simulink model "MPCFollower"  (R2024a)
settings: Solver=FixedStepAuto  StartTime=0.0  StopTime=inf  RelTol=1e-3
undefined symbols (not defined in the file or in its folder): maxLocalPathLen, maxRefPathLen, nlobjTracking
libraries: roshelperlib x2, mpclib x1
settings Model: Creator=cstabile  LastModifiedBy=cstabile

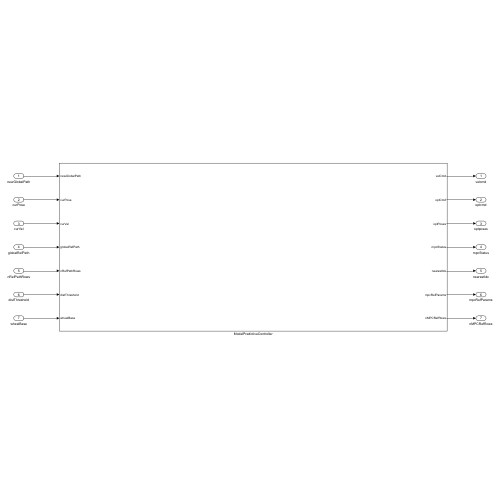
[thumbnail: Simulink's stored preview of the top-level diagram]
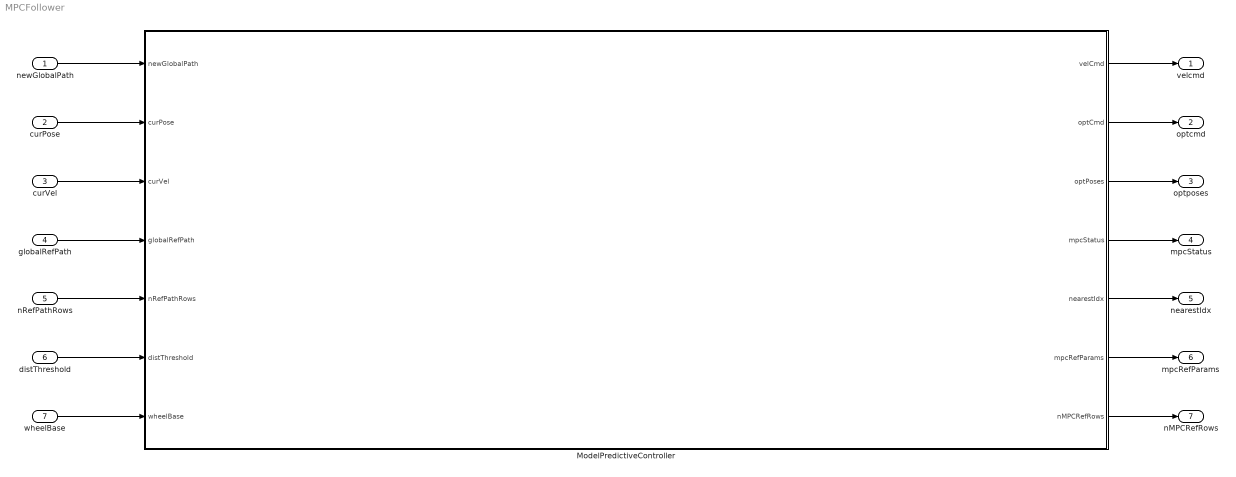
== system MPCFollower ==
  newGlobalPath : Inport  PortDimensions=1
  curPose : Inport  Port=2  PortDimensions=[1 3]
  curVel : Inport  Port=3  PortDimensions=[1 2]
  globalRefPath : Inport  Port=4  PortDimensions=[maxRefPathLen 3]
  nRefPathRows : Inport  Port=5
  distThreshold : Inport  Port=6
  wheelBase : Inport  Port=7
  ModelPredictiveController : Subsystem
  velcmd : Outport  PortDimensions=[1 2]
  optcmd : Outport  Port=2  PortDimensions=[nlobjTracking.PredictionHorizon+1 2]
  optposes : Outport  Port=3  PortDimensions=[nlobjTracking.PredictionHorizon+1 3]
  mpcStatus : Outport  Port=4
  nearestIdx : Outport  Port=5
  mpcRefParams : Outport  Port=6  PortDimensions=[nlobjTracking.PredictionHorizon 3]
  nMPCRefRows : Outport  Port=7  PortDimensions=1
  wires:
  newGlobalPath/1 -> ModelPredictiveController/1(newGlobalPath)
  curPose/1 -> ModelPredictiveController/2(curPose)
  ModelPredictiveController/1(velCmd) -> velcmd/1
  distThreshold/1 -> ModelPredictiveController/6(distThreshold)
  curVel/1 -> ModelPredictiveController/3(curVel)
  globalRefPath/1 -> ModelPredictiveController/4(globalRefPath)
  nRefPathRows/1 -> ModelPredictiveController/5(nRefPathRows)
  wheelBase/1 -> ModelPredictiveController/7(wheelBase)
  ModelPredictiveController/3(optPoses) -> optposes/1
  ModelPredictiveController/2(optCmd) -> optcmd/1
  ModelPredictiveController/5(nearestIdx) -> nearestIdx/1
  ModelPredictiveController/4(mpcStatus) -> mpcStatus/1
  ModelPredictiveController/6(mpcRefParams) -> mpcRefParams/1
  ModelPredictiveController/7(nMPCRefRows) -> nMPCRefRows/1

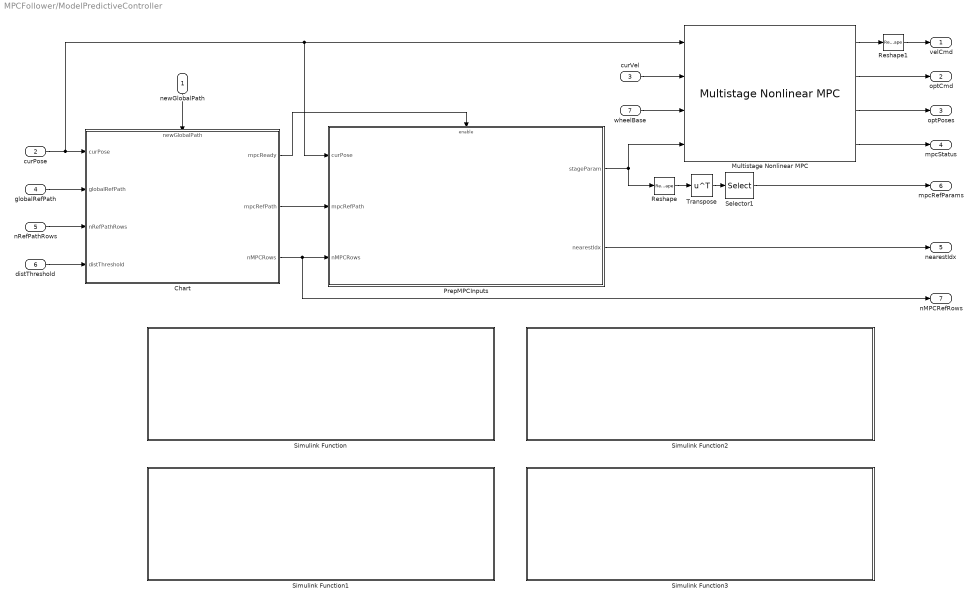
== system MPCFollower/ModelPredictiveController ==
  newGlobalPath : Inport
  curPose : Inport  Port=2  PortDimensions=[1 3]
  curVel : Inport  Port=3
  globalRefPath : Inport  Port=4  PortDimensions=[maxRefPathLen 3]
  nRefPathRows : Inport  Port=5
  distThreshold : Inport  Port=6
  wheelBase : Inport  Port=7
  Chart : Stateflow chart  TreatAsAtomicUnit=on
      settings: PortSchema="{\"entries\":[{\"content\":{\"sides\":[{\"content\":{\"connectorIds\":[\"In2\",\"In3\",\"In4\",\"In5\"]},\"type\":\"ConnectorPlacement.EquallySpacedRectSide\",\"uuid\":\"d330c18e-78c4-4446-bef4-6c07f5901eab\"},{\"content\":{\"connectorIds\":[\"Out1\",\"Out2\",\"Out3\"],\"side\":\"RIGHT\"},\"type\":\"ConnectorPlacement.EquallySpacedRectSide\",\"uuid\":\"b290a02e-6c58-4d00-b488-7afeab83322a\"},{\"content\":{\"connectorIds\":[\"In1\"],\"side\":\"TOP\"},\"type\":\"ConnectorPlacement.EquallySpacedRectSide\",\"uuid\":\"5cf05c0e-e546-4e08-b885-e292e35119c9\"}]},\"type\":\"ConnectorPlacement.EquallySpacedConnector\",\"uuid\":\"c70a4d9b-d7d3-4706-8fc9-b9f30a67664a\"}],\"packageUris\":[\"http://schema.mathworks.com/mf0/Connector/R2020b\"],\"version\":\"1.0\"}"
  Multistage Nonlinear MPC : mpclib/Multistage Nonlinear MPC  nlmpcobj=nlobjTracking  UseObjectTs=on  TsControl=-1  UseMEX=off  mexname=pathFollowingMPCMex  md_enabled=off  stateparam_enabled=on  stageparam_enabled=on  cost_enabled=off  mvseq_enabled=on  stateseq_enabled=on  slack_enabled=off  status_enabled=on  mv_min=off  mv_max=off  mvrate_min=off  mvrate_max=off  state_min=off  state_max=off  terminal_state=off  nlp_initialize=off
  PrepMPCInputs : Subsystem
  Reshape : Reshape  OutputDimensionality=Customize  OutputDimensions=[4,11]
  Reshape1 : Reshape  OutputDimensionality=Row vector (2-D)
  Selector1 : Selector  NumberOfDimensions=2  InputPortWidth=3  IndexOptions=Index vector (dialog),Index vector (dialog)  Indices=2:11,1:3  OutputSizes=1,1
  Simulink Function : Subsystem  TreatAsAtomicUnit=on
  Simulink Function1 : Subsystem  TreatAsAtomicUnit=on
  Simulink Function2 : Subsystem  TreatAsAtomicUnit=on
  Simulink Function3 : Subsystem  TreatAsAtomicUnit=on
  Transpose : Math  Operator=transpose
  velCmd : Outport  PortDimensions=[1 2]
  optCmd : Outport  Port=2
  optPoses : Outport  Port=3
  mpcStatus : Outport  Port=4
  nearestIdx : Outport  Port=5
  mpcRefParams : Outport  Port=6
  nMPCRefRows : Outport  Port=7
  wires:
  curPose/1 -> Multistage Nonlinear MPC/1, PrepMPCInputs/1(curPose), Chart/2(curPose)
  wheelBase/1 -> Multistage Nonlinear MPC/3
  Multistage Nonlinear MPC/2 -> optCmd/1
  Multistage Nonlinear MPC/1 -> Reshape1/1
  distThreshold/1 -> Chart/5(distThreshold)
  Multistage Nonlinear MPC/3 -> optPoses/1
  Multistage Nonlinear MPC/4 -> mpcStatus/1
  curVel/1 -> Multistage Nonlinear MPC/2
  globalRefPath/1 -> Chart/3(globalRefPath)
  nRefPathRows/1 -> Chart/4(nRefPathRows)
  Reshape/1 -> Transpose/1
  Transpose/1 -> Selector1/1
  Selector1/1 -> mpcRefParams/1
  newGlobalPath/1 -> Chart/1(newGlobalPath)
  PrepMPCInputs/1(stageParam) -> Reshape/1, Multistage Nonlinear MPC/4
  Chart/2(mpcRefPath) -> PrepMPCInputs/2(mpcRefPath)
  Chart/3(nMPCRows) -> nMPCRefRows/1, PrepMPCInputs/3(nMPCRows)
  PrepMPCInputs/2(nearestIdx) -> nearestIdx/1
  Chart/1(mpcReady) -> PrepMPCInputs/Enable
  Reshape1/1 -> velCmd/1

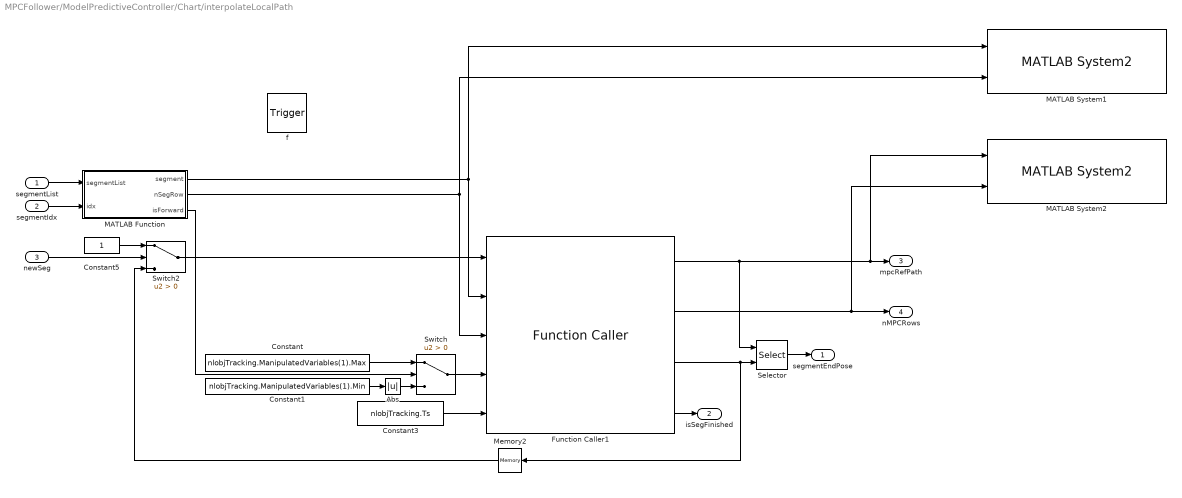
== system MPCFollower/ModelPredictiveController/Chart/interpolateLocalPath ==
  segmentList : Inport  OutDataTypeStr=Bus: mpcPathList_fixed_bus  PortDimensions=1
  segmentIdx : Inport  Port=2  OutDataTypeStr=double  PortDimensions=1
  newSeg : Inport  Port=3  OutDataTypeStr=boolean  PortDimensions=1
  f : TriggerPort  TriggerType=function-call  VariantControl=(inherit)
      settings: CopyFcn=Stateflow.SLINSF.SimulinkMan.removeBlockPreDeleteFcn  PreDeleteFcn=Stateflow.SLINSF.SimulinkMan.unsafePredeleteFcn
  Abs : Abs  SaturateOnIntegerOverflow=off
  Constant : Constant  Value=nlobjTracking.ManipulatedVariables(1).Max
  Constant1 : Constant  Value=nlobjTracking.ManipulatedVariables(1).Min
  Constant3 : Constant  Value=nlobjTracking.Ts
  Constant5 : Constant
  Function Caller1 : FunctionCaller  FunctionPrototype=[localRefPath,nRows,lastIdx,isSegFinished] = arcInterpolateSegment(initIdx,segmentPoses,nSegRows,vNominal,timestep)  InputArgumentSpecifications=<Enter example>  OutputArgumentSpecifications=<Enter example>
  MATLAB Function : MATLAB Function  TreatAsAtomicUnit=on
  MATLAB System1 : roshelperlib/MATLAB System2  VisualizationParameters={'m','LineWidth',4}  PlotType=Line  DisplayVisual=on  SimulateUsing=Interpreted execution
  MATLAB System2 : roshelperlib/MATLAB System2  VisualizationParameters={'r:','LineWidth',3}  PlotType=Line  DisplayVisual=on  SimulateUsing=Interpreted execution
  Memory2 : Memory  InheritSampleTime=on
  Selector : Selector  NumberOfDimensions=2  InputPortWidth=3  IndexOptions=Index vector (port),Select all  Indices=[1 3],1  OutputSizes=1,1
  Switch : Switch  Criteria=u2 > Threshold  SaturateOnIntegerOverflow=off  InputSameDT=off
  Switch2 : Switch  Criteria=u2 > Threshold  SaturateOnIntegerOverflow=off  InputSameDT=off
  segmentEndPose : Outport
  isSegFinished : Outport  Port=2
  mpcRefPath : Outport  Port=3
  nMPCRows : Outport  Port=4
  wires:
  Switch2/1 -> Function Caller1/1
  Constant1/1 -> Abs/1
  Function Caller1/2 -> MATLAB System2/2, nMPCRows/1
  Function Caller1/3 -> Selector/2, Memory2/1
  Constant/1 -> Switch/1
  Switch/1 -> Function Caller1/4
  Selector/1 -> segmentEndPose/1
  Function Caller1/4 -> isSegFinished/1
  segmentList/1 -> MATLAB Function/1(segmentList)
  MATLAB Function/2(nSegRow) -> Function Caller1/3, MATLAB System1/2
  Constant5/1 -> Switch2/1
  segmentIdx/1 -> MATLAB Function/2(idx)
  MATLAB Function/3(isForward) -> Switch/2
  Constant3/1 -> Function Caller1/5
  Function Caller1/1 -> MATLAB System2/1, mpcRefPath/1, Selector/1
  MATLAB Function/1(segment) -> Function Caller1/2, MATLAB System1/1
  Memory2/1 -> Switch2/3
  newSeg/1 -> Switch2/2
  Abs/1 -> Switch/3

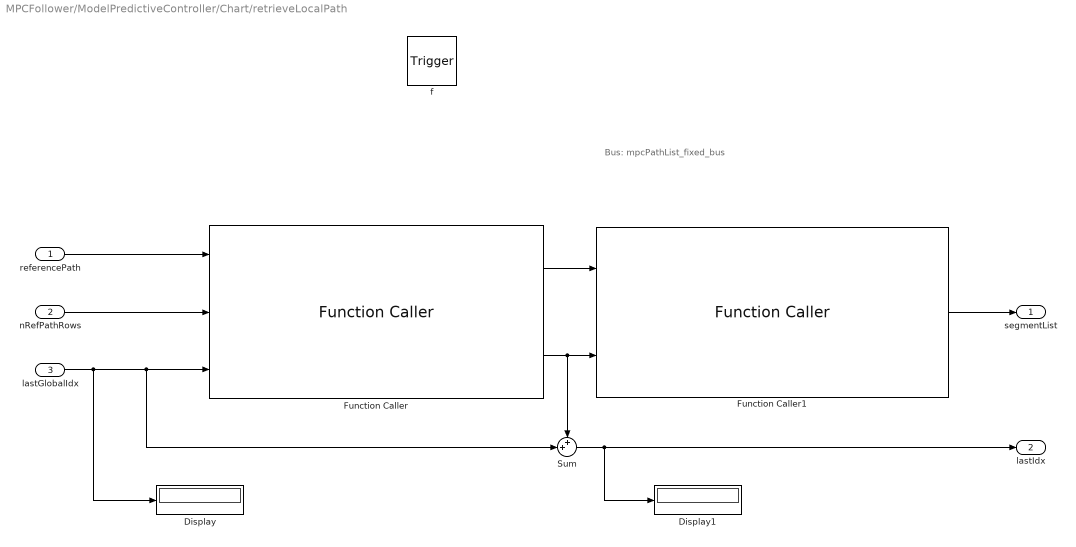
== system MPCFollower/ModelPredictiveController/Chart/retrieveLocalPath ==
  note: Bus: mpcPathList_fixed_bus
  referencePath : Inport  OutDataTypeStr=double  PortDimensions=[maxRefPathLen 3]
  nRefPathRows : Inport  Port=2  OutDataTypeStr=double  PortDimensions=1
  lastGlobalIdx : Inport  Port=3  OutDataTypeStr=double  PortDimensions=1
  f : TriggerPort  TriggerType=function-call  VariantControl=(inherit)
      settings: CopyFcn=Stateflow.SLINSF.SimulinkMan.removeBlockPreDeleteFcn  PreDeleteFcn=Stateflow.SLINSF.SimulinkMan.unsafePredeleteFcn
  Display : Display
  Display1 : Display
  Function Caller : FunctionCaller  FunctionPrototype=[localRefPath,nLocalRows] = getLocalPath(referencePath,nRefPathRows,curGlobalIdx)  InputArgumentSpecifications=<Enter example>  OutputArgumentSpecifications=<Enter example>
  Function Caller1 : FunctionCaller  FunctionPrototype=segmentList = path2segments(referencePath,nLocalRows)  InputArgumentSpecifications=<Enter example>  OutputArgumentSpecifications=<Enter example>
  Sum : Sum  Inputs=++|
  segmentList : Outport  OutDataTypeStr=Bus: mpcPathList_fixed_bus  PortDimensions=1
  lastIdx : Outport  Port=2  OutDataTypeStr=double  PortDimensions=1
  wires:
  lastGlobalIdx/1 -> Display/1, Sum/2, Function Caller/3
  Function Caller/1 -> Function Caller1/1
  nRefPathRows/1 -> Function Caller/2
  referencePath/1 -> Function Caller/1
  Function Caller/2 -> Sum/1, Function Caller1/2
  Sum/1 -> Display1/1, lastIdx/1
  Function Caller1/1 -> segmentList/1

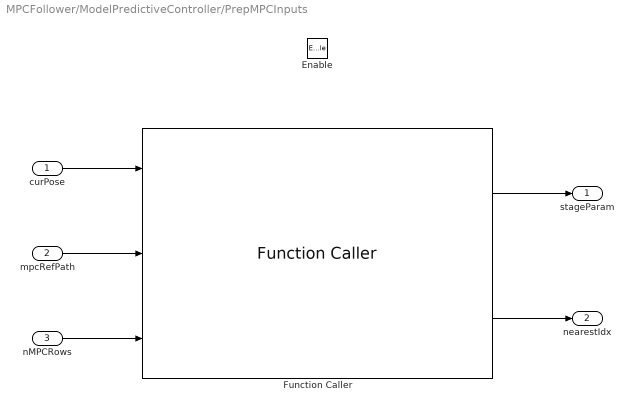
== system MPCFollower/ModelPredictiveController/PrepMPCInputs ==
  curPose : Inport
  mpcRefPath : Inport  Port=2
  nMPCRows : Inport  Port=3
  Enable : EnablePort  StatesWhenEnabling=reset
  Function Caller : FunctionCaller  FunctionPrototype=[stageParam,idx] = generateMPCReferenceStates(curPose,refPath,nRefPathRows)  InputArgumentSpecifications=<Enter example>  OutputArgumentSpecifications=<Enter example>
  stageParam : Outport
  nearestIdx : Outport  Port=2
  wires:
  Function Caller/1 -> stageParam/1
  nMPCRows/1 -> Function Caller/3
  curPose/1 -> Function Caller/1
  mpcRefPath/1 -> Function Caller/2
  Function Caller/2 -> nearestIdx/1

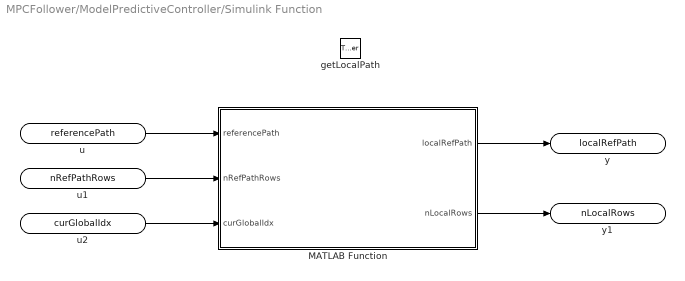
== system MPCFollower/ModelPredictiveController/Simulink Function ==
  getLocalPath : TriggerPort  TriggerType=function-call  IsSimulinkFunction=on  FunctionName=getLocalPath  VariantControl=(inherit)
  MATLAB Function : MATLAB Function  TreatAsAtomicUnit=on  mask{maxPathLength=maxRefPathLen, maxLocalLength=maxLocalPathLen}
      mask prompts: maxPathLength "Max Path Length"; maxLocalLength "Max Local Path Length"
  u : ArgIn  DisableCoverage=on  PortDimensions=[maxRefPathLen 3]  ArgumentName=referencePath
  u1 : ArgIn  DisableCoverage=on  Port=2  ArgumentName=nRefPathRows
  u2 : ArgIn  DisableCoverage=on  Port=3  ArgumentName=curGlobalIdx
  y : ArgOut  DisableCoverage=on  PortDimensions=[maxLocalPathLen 3]  ArgumentName=localRefPath
  y1 : ArgOut  DisableCoverage=on  Port=2  ArgumentName=nLocalRows
  wires:
  MATLAB Function/1(localRefPath) -> y/1
  MATLAB Function/2(nLocalRows) -> y1/1
  u/1 -> MATLAB Function/1(referencePath)
  u2/1 -> MATLAB Function/3(curGlobalIdx)
  u1/1 -> MATLAB Function/2(nRefPathRows)

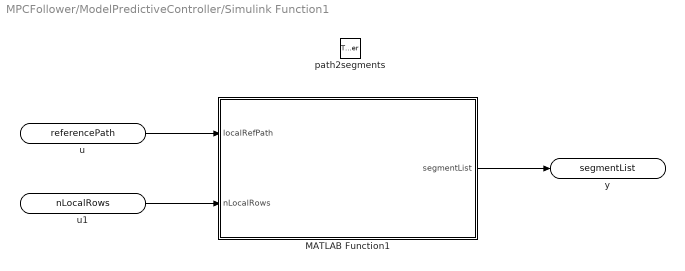
== system MPCFollower/ModelPredictiveController/Simulink Function1 ==
  path2segments : TriggerPort  TriggerType=function-call  IsSimulinkFunction=on  FunctionName=path2segments  VariantControl=(inherit)
  MATLAB Function1 : MATLAB Function  TreatAsAtomicUnit=on  mask{maxPathLength=maxRefPathLen, maxLocalLength=maxLocalPathLen}
      mask prompts: maxPathLength "Max Path Length"; maxLocalLength "Max Local Path Length"
  u : ArgIn  DisableCoverage=on  PortDimensions=[maxLocalPathLen 3]  ArgumentName=referencePath
  u1 : ArgIn  DisableCoverage=on  Port=2  ArgumentName=nLocalRows
  y : ArgOut  DisableCoverage=on  OutDataTypeStr=Bus: mpcPathList_fixed_bus  ArgumentName=segmentList
  wires:
  MATLAB Function1/1(segmentList) -> y/1
  u/1 -> MATLAB Function1/1(localRefPath)
  u1/1 -> MATLAB Function1/2(nLocalRows)

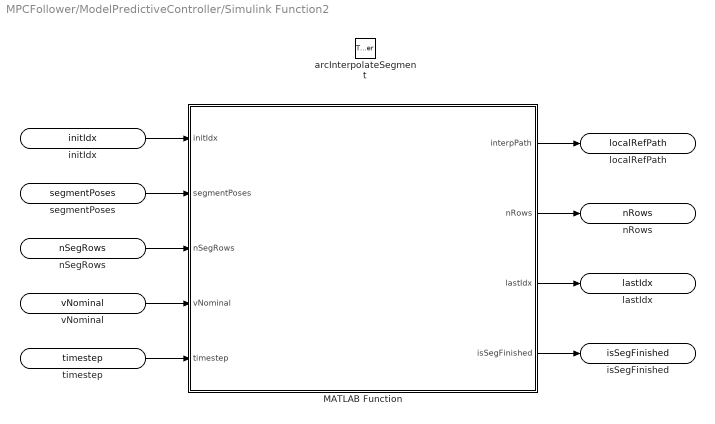
== system MPCFollower/ModelPredictiveController/Simulink Function2 ==
  arcInterpolateSegment : TriggerPort  TriggerType=function-call  IsSimulinkFunction=on  FunctionName=arcInterpolateSegment  VariantControl=(inherit)
  MATLAB Function : MATLAB Function  TreatAsAtomicUnit=on  mask{maxPathLength=maxLocalPathLen}
      mask prompts: maxPathLength "Max Path Length"
  initIdx : ArgIn  DisableCoverage=on  ArgumentName=initIdx
  segmentPoses : ArgIn  DisableCoverage=on  Port=2  PortDimensions=[maxLocalPathLen 3]  ArgumentName=segmentPoses
  nSegRows : ArgIn  DisableCoverage=on  Port=3  ArgumentName=nSegRows
  vNominal : ArgIn  DisableCoverage=on  Port=4  ArgumentName=vNominal
  timestep : ArgIn  DisableCoverage=on  Port=5  ArgumentName=timestep
  localRefPath : ArgOut  DisableCoverage=on  PortDimensions=[maxLocalPathLen 3]  ArgumentName=localRefPath
  nRows : ArgOut  DisableCoverage=on  Port=2  ArgumentName=nRows
  lastIdx : ArgOut  DisableCoverage=on  Port=3  ArgumentName=lastIdx
  isSegFinished : ArgOut  DisableCoverage=on  Port=4  OutDataTypeStr=boolean  ArgumentName=isSegFinished
  wires:
  segmentPoses/1 -> MATLAB Function/2(segmentPoses)
  initIdx/1 -> MATLAB Function/1(initIdx)
  vNominal/1 -> MATLAB Function/4(vNominal)
  timestep/1 -> MATLAB Function/5(timestep)
  MATLAB Function/1(interpPath) -> localRefPath/1
  MATLAB Function/3(lastIdx) -> lastIdx/1
  MATLAB Function/4(isSegFinished) -> isSegFinished/1
  MATLAB Function/2(nRows) -> nRows/1
  nSegRows/1 -> MATLAB Function/3(nSegRows)

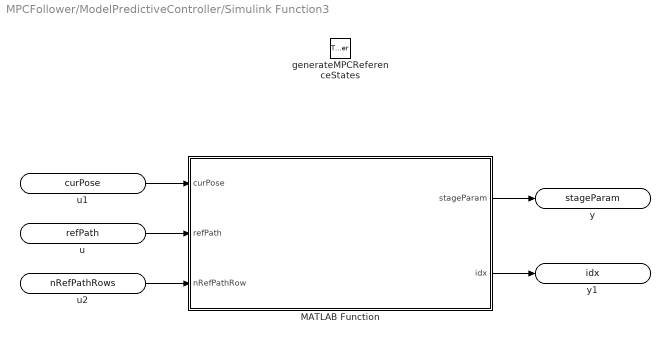
== system MPCFollower/ModelPredictiveController/Simulink Function3 ==
  generateMPCReferenceStates : TriggerPort  TriggerType=function-call  IsSimulinkFunction=on  FunctionName=generateMPCReferenceStates  VariantControl=(inherit)
  MATLAB Function : MATLAB Function  TreatAsAtomicUnit=on  mask{predictionHorizon=nlobjTracking.PredictionHorizon}
      mask prompts: predictionHorizon "MPC Prediction Horizon"
  u1 : ArgIn  DisableCoverage=on  PortDimensions=[1 3]  ArgumentName=curPose
  u : ArgIn  DisableCoverage=on  Port=2  PortDimensions=[maxLocalPathLen 3]  ArgumentName=refPath
  u2 : ArgIn  DisableCoverage=on  Port=3  ArgumentName=nRefPathRows
  y : ArgOut  DisableCoverage=on  PortDimensions=(nlobjTracking.PredictionHorizon+1)*4  ArgumentName=stageParam
  y1 : ArgOut  DisableCoverage=on  Port=2  ArgumentName=idx
  wires:
  u/1 -> MATLAB Function/2(refPath)
  u1/1 -> MATLAB Function/1(curPose)
  u2/1 -> MATLAB Function/3(nRefPathRow)
  MATLAB Function/1(stageParam) -> y/1
  MATLAB Function/2(idx) -> y1/1

== matlab function MPCFollower/ModelPredictiveController/Simulink Function/MATLAB Function ==
  data: referencePath input size=[maxPathLength 3]; nRefPathRows input; localRefPath output size=[maxLocalLength 3]; curGlobalIdx input; nLocalRows output; maxPathLength parameter; maxLocalLength parameter
function [localRefPath,nLocalRows] = getLocalPath(referencePath,nRefPathRows,curGlobalIdx, maxPathLength, maxLocalLength)
%getLocalPath Extract upcoming N poses from input path

localRefPath = zeros(maxLocalLength,3);
nLocalRows = min(nRefPathRows-(curGlobalIdx-1),maxLocalLength);
localRefPath(1:nLocalRows,:) = referencePath(curGlobalIdx:(curGlobalIdx+nLocalRows-1),:);

== matlab function MPCFollower/ModelPredictiveController/Simulink Function3/MATLAB Function ==
  data: curPose input; stageParam output; refPath input; nRefPathRow input; idx output; predictionHorizon parameter
function [stageParam,idx] = generateMPCReferenceStates(curPose, refPath, nRefPathRow, predictionHorizon)
%generateMPCReferenceStates Extract reference poses for MPC controller given initial state and prediction horizon
    [stageParam,idx] = exampleHelperGenerateMPCReferenceSegment(curPose,refPath(1:nRefPathRow,:),predictionHorizon);
end

== matlab function MPCFollower/ModelPredictiveController/Simulink Function1/MATLAB Function1 ==
  data: localRefPath input size=[maxLocalPathLen 3]; nLocalRows input; segmentList output Bus: mpcPathList_fixed_bus; maxRefPathLen parameter; maxLocalPathLen parameter
function segmentList = path2segments(localRefPath,nLocalRows,maxRefPathLen,maxLocalPathLen)
%path2segments Identify uni-directional list of segments

% Break refPath into pieces
[segArray,pivotIdx,nSeg] = exampleHelperFindPivots(localRefPath(1:nLocalRows,:));
segmentList = exampleHelperEncodeBus(segArray,maxRefPathLen,maxLocalPathLen,Widths=size(localRefPath,2));

== matlab function MPCFollower/ModelPredictiveController/Simulink Function2/MATLAB Function ==
  data: initIdx input; segmentPoses input; nSegRows input; interpPath output; nRows output; vNominal input; timestep input; lastIdx output; isSegFinished output; maxPathLength parameter
function [interpPath,nRows,lastIdx,isSegFinished] = arcInterpolateSegment(initIdx,segmentPoses,nSegRows,vNominal,timestep,maxPathLength)
    fullyInterpedPath = exampleHelperEvenlyInterpSegment(segmentPoses(1:nSegRows,:),vNominal,timestep);
    lastIdx = initIdx+size(fullyInterpedPath,1)-1;
    if lastIdx <= maxPathLength
        isSegFinished = true;
    else
        lastIdx = initIdx+maxPathLength-1;
        isSegFinished = false;
    end
    nRows = 1+lastIdx-initIdx;
    interpPath = zeros(maxPathLength,3);
    interpPath(1:nRows,:) = fullyInterpedPath(initIdx:lastIdx,:);
end

== stateflow chart MPCFollower/ModelPredictiveController/Chart ==
  state WaitForPath
    mpcReady = 0;
  state Running
    Running -> (junction 4) [order 1] : {
        | vSegment = segGoal(:)-curPose(:);
        | vGoal = goalPose(:)-curPose(:);
        | }
    (junction 4) -> (junction 73) [order 1] : [norm(vSegment(1:2),2) <= distThreshold]
    (junction 73) -> (junction 8) [order 1] : [isSegFinished]
    (junction 8) -> (junction 12) [order 1] : [curSegIdx == nSeg]
    (junction 12) -> (junction 122) [order 1] : [norm(vGoal(1:2),2) <= distThreshold]
        | {mpcReady=0;}
    (junction 73) -> (junction 65) [order 2]
    (junction 4) -> (junction 10) [order 2]
    (junction 8) -> (junction 65) [order 2]
    (junction 12) -> (junction 15) [order 2] : {
        | curSegIdx=0;
        | [segmentList,lastIdx] = retrieveLocalPath(globalRefPath,nRefPathRows,lastIdx);
        | nSeg = segmentList.States_N;
        | }
    (junction 15) -> (junction 65)
    (junction 65) -> (junction 62) : {
        | curSegIdx = curSegIdx+1;
        | [segGoal,isSegFinished,mpcRefPath,nMPCRows] = ...
        |  interpolateLocalPath(segmentList, curSegIdx, isSegFinished);
        | }
    (junction 10) -> (junction 108) : {mpcReady = 1;}
    (junction 62) -> (junction 10)
  state [segmentList,lastIdx] = retrieveLocalPath(referencePath,nRefPathRows,lastGlobalIdx) [function]
  state [segmentEndPose,isSegFinished,mpcRefPath,nMPCRows] = interpolateLocalPath(segmentList,segmentIdx,newSeg) [function]
  (default) -> (junction 110) : {newGlobalPathInternal = newGlobalPath;}
  WaitForPath -> (junction 110)
  (junction 110) -> (junction 93) [order 1] : [newGlobalPathInternal]
  (junction 110) -> WaitForPath [order 2] : {newGlobalPathInternal = newGlobalPath;}
  Running -> (junction 110) [order 2] : [newGlobalPath]
  (junction 93) -> Running : {
      | newGlobalPathInternal = 0;
      | curSegIdx=1;
      | lastIdx = 1;
      | [segmentList,lastIdx] = retrieveLocalPath(globalRefPath,nRefPathRows,lastIdx);
      | nSeg = segmentList.States_N;
      | goalPose = globalRefPath(nRefPathRows,:);
      | isSegFinished = true;
      | [segGoal,isSegFinished,mpcRefPath,nMPCRows] = interpolateLocalPath(segmentList, curSegIdx, isSegFinished);
      | vGoal = goalPose(:)-curPose(:);
      | }
  Running -> WaitForPath [order 1] : [norm(vGoal(1:2),2) <= distThreshold && curSegIdx == nSeg]
      | {newGlobalPathInternal = newGlobalPath;}
  data: referencePath function_input double size=[maxRefPathLen 3]; nRefPathRows function_input double size=1; lastGlobalIdx function_input double size=1; segmentList function_output Bus: mpcPathList_fixed_bus size=1; lastIdx function_output double size=1; segmentList function_input Bus: mpcPathList_fixed_bus size=1; segmentIdx function_input double size=1; segmentEndPose function_output; isSegFinished function_output; mpcRefPath function_output; nMPCRows function_output; newSeg function_input boolean size=1; mpcReady output; newGlobalPath input; curPose input; globalRefPath input double size=[maxRefPathLen 3]; nRefPathRows input; distThreshold input; segmentList local Bus: mpcPathList_fixed_bus size=1; lastIdx local; mpcRefPath output size=[maxLocalPathLen 3]; nMPCRows output; segGoal local; isSegFinished local; curSegIdx local; nSeg local; goalPose local; vGoal local; vSegment local; newGlobalPathInternal local

== matlab function MPCFollower/ModelPredictiveController/Chart/interpolateLocalPath/MATLAB Function ==
  data: segmentList input; segment output size=[maxLocalPathLen 3]; idx input; maxLocalPathLen parameter; nSegRow output; isForward output
function [segment,nSegRow,isForward] = getSegment(segmentList,idx,maxLocalPathLen)
%getSegment Retrieve segment from list and determine motion direction
    segment = zeros(maxLocalPathLen,3);
    ptIdx = segmentList.StatesIndices(idx,:);
    nSegRow = diff(ptIdx)+1;
    seg = segmentList.States(ptIdx(1):ptIdx(2),:);
    vHeading = [cos(seg(:,3)) sin(seg(:,3))];
    vDirection = normalize(diff(seg(:,1:2)),2,'norm');
    isForward = sum(vHeading(1:end-1,:).*vDirection,"all") > 0;
    segment(1:nSegRow,:) = seg;
end
